simulink model "SiMoDronesMK"  (R2022a)
settings: Solver=FixedStepAuto  StartTime=0.0  StopTime=60  FixedStep=0.005  MaxStep=1e-3  MinStep=5e-5  RelTol=1e-5  AbsTol=1e-5  EnableMultiTasking=on
StopFcn:
  | save log.mat
  | [px4,optitrack,control,simulink]=traite_data_full('log.mat');
  | plot_data;
values from neighbouring files (symbols this model uses):
  aero =     [log.mat]
  drone =     [log.mat]
  dT_px4_udp = 0.02    [SimulationStartupScript.m]    (also in log.mat)
  dT_udp = 0.02    [SimulationStartupScript.m]    (also in log.mat)
  dT_udp_px4 = 0.02    [SimulationStartupScript.m]    (also in log.mat)
  Iload_UAVaxis = [0.00408625  0  0; 0  0.00408625  0; 0  0  8.625e-05]    [log.mat]
  init_state =     [log.mat]
  kpx = 1    [log.mat]
  kvx = 0.35    [log.mat]
  mass = 0.207    [log.mat]
  measure =     [log.mat]
  motor =     [log.mat]
  noisetrigger = 0    [log.mat]
  regul =     [log.mat]
  tdrop = 30    [SimulationStartupScript.m]    (also in log.mat)
  Te = 2e-2    (= 0.02)    [SimulationStartupScript.m]    (also in log.mat)
  th0 = 0.45    [log.mat]
  Ts_px4 = 5e-3    (= 0.005)    [SimulationStartupScript.m]    (also in log.mat)
undefined symbols (not defined in the file or in its folder): DiscIntNeverNeededParam, frame_t, gcbh, sigbuilder_block, sldrt_modeswitch, Standard_Devices, UDP_Protocol
libraries: simulink x11, orocomplib x9, vrlib x5, sldrtlib x4, sharedtransform x3, shared6dofsys x2, sharedutil x1, shared6dof x1, lib_isae_drones x1, simulink_need_slupdate x1, aerolibanimutils x1
(part 3 of 3)

== system SiMoDronesMK/Mass Change Model/Model/Quad rotor model1/Modèle Moments/Calcul Trainée Angulaire ==
  In1 : Inport
  Demux : Demux  Outputs=3
  Demux1 : Demux  Outputs=3
  Gain : Gain  Gain=-1
  Gain2 : Gain  Gain=.5
  Gain3 : Gain  Gain=-1
  Gain4 : Gain  Gain=-1
  Gain5 : Gain  Gain=L
  In2 : InportShadow
  Math Function : Math  Operator=square  SignedPower=on
  Mux2 : Mux  Inputs=3
  Product{1..2,4..5} (4 alike) : Product  RndMeth=Zero
  Product3 : Product  Inputs=3  RndMeth=Zero
  Sign1 : Signum
  Sign2 : Signum
  Sign3 : Signum
  Surface Active : Constant  Value=S_trainee_pqr  SampleTime=0
  density : Constant  Value=rho  SampleTime=0
  dragCoeff : Constant  Value=C_trainee  SampleTime=0
  Out1 : Outport
  wires:
  Surface Active/1 -> Product3/2
  Product3/1 -> Demux/1
  Math Function/1 -> Product4/1
  Gain4/1 -> Mux2/3
  Gain3/1 -> Mux2/2
  Gain/1 -> Mux2/1
  Demux/3 -> Product5/2
  Demux/2 -> Product2/2
  Demux/1 -> Product1/2
  Sign3/1 -> Product5/1
  Sign1/1 -> Product2/1
  Sign2/1 -> Product1/1
  Demux1/3 -> Sign3/1
  Demux1/2 -> Sign1/1
  Demux1/1 -> Sign2/1
  In2/1 -> Demux1/1  "p q r"
  Product1/1 -> Gain/1
  Product2/1 -> Gain3/1
  Product5/1 -> Gain4/1
  density/1 -> Gain2/1
  dragCoeff/1 -> Product3/3  "Cd"
  Product4/1 -> Product3/1
  Gain2/1 -> Product4/2
  In1/1 -> Math Function/1  "p q r"
  Gain5/1 -> Out1/1  "Trainee_angulaires_Rb"
  Mux2/1 -> Gain5/1

== system SiMoDronesMK/Measurement block /Measure /optitrack/XYZ optitrack/1er ordre ==
  x : Inport
  Gain1 : Gain  Gain=1/tr5
  Gain2 : Gain  Gain=K
  Integrator : Integrator  InitialCondition=init_inte
  Sum4 : Sum  Inputs=|+-
  x_retard : Outport
  wires:
  Gain2/1 -> x_retard/1
  x/1 -> Sum4/1
  Sum4/1 -> Gain1/1
  Integrator/1 -> Sum4/2, Gain2/1
  Gain1/1 -> Integrator/1

== system SiMoDronesMK/Measurement block /Measure /optitrack/XYZ optitrack/1er ordre1 ==
  y : Inport
  Gain1 : Gain  Gain=1/tr5
  Gain2 : Gain  Gain=K
  Integrator : Integrator  InitialCondition=init_inte
  Sum4 : Sum  Inputs=|+-
  y_retard : Outport
  wires:
  Gain1/1 -> Integrator/1
  Integrator/1 -> Gain2/1, Sum4/2
  Sum4/1 -> Gain1/1
  y/1 -> Sum4/1
  Gain2/1 -> y_retard/1

== system SiMoDronesMK/Measurement block /Measure /optitrack/XYZ optitrack/1er ordre2 ==
  z : Inport
  Gain1 : Gain  Gain=1/tr5
  Gain2 : Gain  Gain=K
  Integrator : Integrator  InitialCondition=init_inte
  Sum4 : Sum  Inputs=|+-
  z_retard : Outport
  wires:
  Gain2/1 -> z_retard/1
  z/1 -> Sum4/1
  Sum4/1 -> Gain1/1
  Integrator/1 -> Sum4/2, Gain2/1
  Gain1/1 -> Integrator/1

== system SiMoDronesMK/Measurement block /Measure /optitrack/XYZ optitrack/Optitrack  V Noise ==
  Band-Limited White Noise3 : simulink/Sources/Band-Limited White Noise  Cov=[measure.noise_power_vit]  Ts=Te  seed=[23341]
  Constant4 : Constant  Value=noisetrigger  OutDataTypeStr=uint8  SampleTime=Te
  Constant5 : Constant  Value=0  OutDataTypeStr=uint8  SampleTime=Te
  Switch1 : Switch  Criteria=u2 > Threshold  SaturateOnIntegerOverflow=off  InputSameDT=off
  Out1 : Outport
  wires:
  Constant5/1 -> Switch1/3
  Constant4/1 -> Switch1/2
  Switch1/1 -> Out1/1
  Band-Limited White Noise3/1 -> Switch1/1

== system SiMoDronesMK/Measurement block /Measure /optitrack/XYZ optitrack/Optitrack XYZ Noise ==
  Band-Limited White Noise1 : simulink/Sources/Band-Limited White Noise  Cov=[measure.noise_power]  Ts=Te  seed=[23341]
  Constant1 : Constant  Value=noisetrigger  OutDataTypeStr=uint8  SampleTime=Te
  Constant3 : Constant  Value=0  OutDataTypeStr=uint8  SampleTime=Te
  Switch : Switch  Criteria=u2 > Threshold  SaturateOnIntegerOverflow=off  InputSameDT=off
  Out1 : Outport
  wires:
  Switch/1 -> Out1/1
  Constant3/1 -> Switch/3
  Band-Limited White Noise1/1 -> Switch/1
  Constant1/1 -> Switch/2

== system SiMoDronesMK/Measurement block /UDP link + Measure/UDP link/Subsystem4/Float ==
  Float : Inport
  " trame1" : Display  Commented=on
  " trame2" : Display  Commented=on
  Demux : Demux  Outputs=2
  Demux1 : Demux
  MATLAB Function : MATLAB Function  TreatAsAtomicUnit=on
  To Workspace11 : ToWorkspace  VariableName=att_tgt_px4_feedback  SampleTime=Te
  To Workspace4 : ToWorkspace  VariableName=pos_vel_optitrack  SampleTime=Te
  To Workspace6 : ToWorkspace  VariableName=batt_info  SampleTime=Te
  To Workspace7 : ToWorkspace  VariableName=att_eul_px4  SampleTime=Te
  To Workspace8 : ToWorkspace  VariableName=imu_pressure_px4  SampleTime=Te
  To Workspace9 : ToWorkspace  VariableName=att_eul_optitrack  SampleTime=Te
  att_eul_px4 : Outport
  pos_vel_optitrack : Outport  Port=2
  att_eul_optitrack : Outport  Port=3
  tag scope: Vbat=global, pos=global, thrust_back=global
  wires:
  MATLAB Function/2(pos_vel) -> To Workspace4/1, Demux/1, pos_vel_optitrack/1
  MATLAB Function/1(att_eul) -> att_eul_px4/1, To Workspace7/1
  Float/1 -> MATLAB Function/1(u)
  MATLAB Function/3(batt_info) -> To Workspace6/1, [Vbat]
  MATLAB Function/5(att_eul_tgt_out) -> " trame2"/1
  MATLAB Function/4(att_eul_tgt_in) -> " trame1"/1
  Demux/1 -> [pos]
  Demux1/4 -> [thrust_back]
  MATLAB Function/7(att_tgt_PX4) -> Demux1/1, To Workspace11/1
  MATLAB Function/6(optitrack_euler) -> att_eul_optitrack/1, To Workspace9/1
  MATLAB Function/10(imu_acc) -> ?
  MATLAB Function/9(imu_static_pressure) -> To Workspace8/1
  MATLAB Function/8(pos_vel_tgt) -> ?

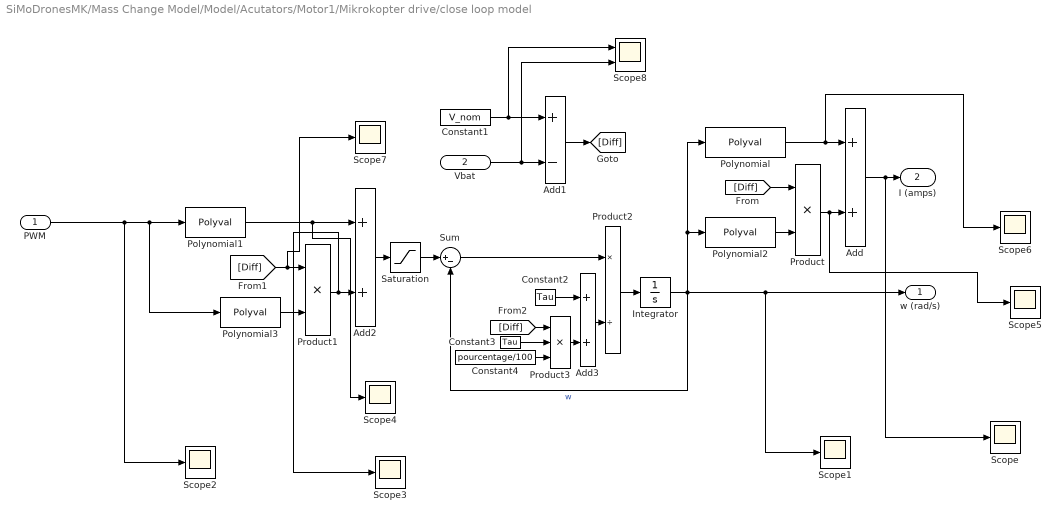
== system SiMoDronesMK/Mass Change Model/Model/Acutators/Motor1/Mikrokopter drive/close loop model ==
  PWM : Inport
  "Vbat " : Inport  Port=2  OutDataTypeStr=double  PortDimensions=1  SampleTime=0
  Add : Sum
  Add1 : Sum  Inputs=+-
  Add2 : Sum
  Add3 : Sum
  Constant1 : Constant  Value=V_nom  SampleTime=-1
  Constant2 : Constant  Value=Tau
  Constant3 : Constant  Value=Tau
  Constant4 : Constant  Value=pourcentage/100
  Integrator : Integrator  InitialCondition=omega_0  LowerSaturationLimit=0
  Polynomial : Polyval  Coefs=coef_w2I
  Polynomial1 : Polyval  Coefs=coef_t2w
  Polynomial2 : Polyval  Coefs=coef_delta_w2I
  Polynomial3 : Polyval  Coefs=coef_delta_t2w
  Product : Product
  Product1 : Product
  Product2 : Product  Inputs=*/
  Product3 : Product  Inputs=***
  Saturation : Saturate  UpperLimit=omega_max  LowerLimit=0
  Scope{,1..7} (8 alike) : Scope
  Scope8 : Scope  NumInputPorts=2
  Sum : Sum  Inputs=|+-
  w (rad/s) : Outport
  I (amps) : Outport  Port=2
  wires:
  Saturation/1 -> Sum/1
  PWM/1 -> Scope2/1, Polynomial1/1, Polynomial3/1
  Integrator/1 -> Scope1/1, w (rad/s)/1, Sum/2, Polynomial2/1, Polynomial/1  "w"
  Sum/1 -> Product2/1
  Polynomial/1 -> Scope6/1, Add/1
  Add/1 -> Scope/1, I (amps)/1
  Add1/1 -> [Diff]
  "Vbat "/1 -> Scope8/2, Add1/2
  Product/1 -> Scope5/1, Add/2
  [Diff] -> Product/1
  Polynomial2/1 -> Product/2
  Polynomial1/1 -> Scope4/1, Add2/1
  Product1/1 -> Scope3/1, Add2/2
  [Diff] -> Scope7/1, Product1/1
  Polynomial3/1 -> Product1/2
  Add2/1 -> Saturation/1
  Product2/1 -> Integrator/1
  Add3/1 -> Product2/2
  Constant2/1 -> Add3/1
  Product3/1 -> Add3/2
  [Diff] -> Product3/1
  Constant3/1 -> Product3/2
  Constant4/1 -> Product3/3
  Constant1/1 -> Scope8/1, Add1/1

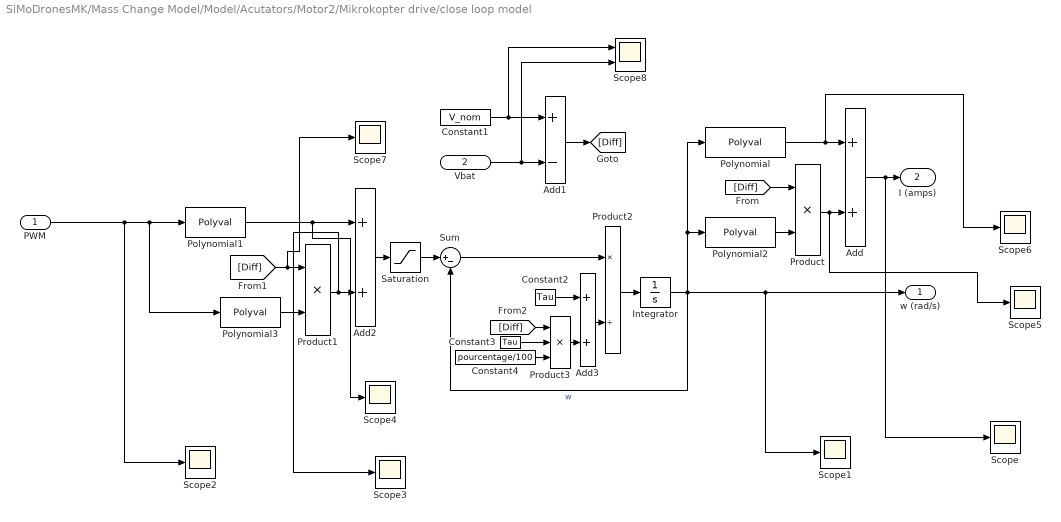
== system SiMoDronesMK/Mass Change Model/Model/Acutators/Motor2/Mikrokopter drive/close loop model ==
  PWM : Inport
  "Vbat " : Inport  Port=2  OutDataTypeStr=double  PortDimensions=1  SampleTime=0
  Add : Sum
  Add1 : Sum  Inputs=+-
  Add2 : Sum
  Add3 : Sum
  Constant1 : Constant  Value=V_nom  SampleTime=-1
  Constant2 : Constant  Value=Tau
  Constant3 : Constant  Value=Tau
  Constant4 : Constant  Value=pourcentage/100
  Integrator : Integrator  InitialCondition=omega_0  LowerSaturationLimit=0
  Polynomial : Polyval  Coefs=coef_w2I
  Polynomial1 : Polyval  Coefs=coef_t2w
  Polynomial2 : Polyval  Coefs=coef_delta_w2I
  Polynomial3 : Polyval  Coefs=coef_delta_t2w
  Product : Product
  Product1 : Product
  Product2 : Product  Inputs=*/
  Product3 : Product  Inputs=***
  Saturation : Saturate  UpperLimit=omega_max  LowerLimit=0
  Scope{,1..7} (8 alike) : Scope
  Scope8 : Scope  NumInputPorts=2
  Sum : Sum  Inputs=|+-
  w (rad/s) : Outport
  I (amps) : Outport  Port=2
  wires:
  Saturation/1 -> Sum/1
  PWM/1 -> Scope2/1, Polynomial1/1, Polynomial3/1
  Integrator/1 -> Scope1/1, w (rad/s)/1, Sum/2, Polynomial2/1, Polynomial/1  "w"
  Sum/1 -> Product2/1
  Polynomial/1 -> Scope6/1, Add/1
  Add/1 -> Scope/1, I (amps)/1
  Add1/1 -> [Diff]
  "Vbat "/1 -> Scope8/2, Add1/2
  Product/1 -> Scope5/1, Add/2
  [Diff] -> Product/1
  Polynomial2/1 -> Product/2
  Polynomial1/1 -> Scope4/1, Add2/1
  Product1/1 -> Scope3/1, Add2/2
  [Diff] -> Scope7/1, Product1/1
  Polynomial3/1 -> Product1/2
  Add2/1 -> Saturation/1
  Product2/1 -> Integrator/1
  Add3/1 -> Product2/2
  Constant2/1 -> Add3/1
  Product3/1 -> Add3/2
  [Diff] -> Product3/1
  Constant3/1 -> Product3/2
  Constant4/1 -> Product3/3
  Constant1/1 -> Scope8/1, Add1/1

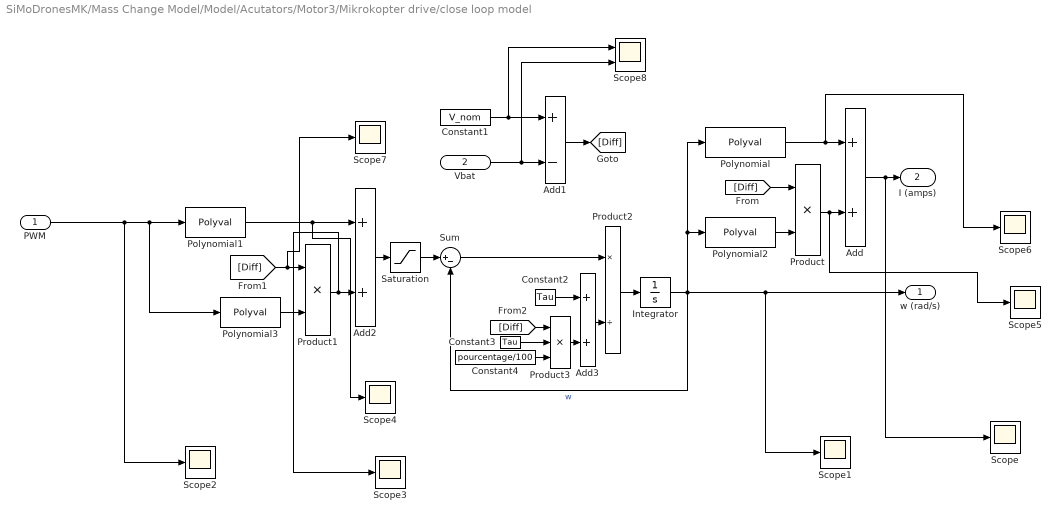
== system SiMoDronesMK/Mass Change Model/Model/Acutators/Motor3/Mikrokopter drive/close loop model ==
  PWM : Inport
  "Vbat " : Inport  Port=2  OutDataTypeStr=double  PortDimensions=1  SampleTime=0
  Add : Sum
  Add1 : Sum  Inputs=+-
  Add2 : Sum
  Add3 : Sum
  Constant1 : Constant  Value=V_nom  SampleTime=-1
  Constant2 : Constant  Value=Tau
  Constant3 : Constant  Value=Tau
  Constant4 : Constant  Value=pourcentage/100
  Integrator : Integrator  InitialCondition=omega_0  LowerSaturationLimit=0
  Polynomial : Polyval  Coefs=coef_w2I
  Polynomial1 : Polyval  Coefs=coef_t2w
  Polynomial2 : Polyval  Coefs=coef_delta_w2I
  Polynomial3 : Polyval  Coefs=coef_delta_t2w
  Product : Product
  Product1 : Product
  Product2 : Product  Inputs=*/
  Product3 : Product  Inputs=***
  Saturation : Saturate  UpperLimit=omega_max  LowerLimit=0
  Scope{,1..7} (8 alike) : Scope
  Scope8 : Scope  NumInputPorts=2
  Sum : Sum  Inputs=|+-
  w (rad/s) : Outport
  I (amps) : Outport  Port=2
  wires:
  Saturation/1 -> Sum/1
  PWM/1 -> Scope2/1, Polynomial1/1, Polynomial3/1
  Integrator/1 -> Scope1/1, w (rad/s)/1, Sum/2, Polynomial2/1, Polynomial/1  "w"
  Sum/1 -> Product2/1
  Polynomial/1 -> Scope6/1, Add/1
  Add/1 -> Scope/1, I (amps)/1
  Add1/1 -> [Diff]
  "Vbat "/1 -> Scope8/2, Add1/2
  Product/1 -> Scope5/1, Add/2
  [Diff] -> Product/1
  Polynomial2/1 -> Product/2
  Polynomial1/1 -> Scope4/1, Add2/1
  Product1/1 -> Scope3/1, Add2/2
  [Diff] -> Scope7/1, Product1/1
  Polynomial3/1 -> Product1/2
  Add2/1 -> Saturation/1
  Product2/1 -> Integrator/1
  Add3/1 -> Product2/2
  Constant2/1 -> Add3/1
  Product3/1 -> Add3/2
  [Diff] -> Product3/1
  Constant3/1 -> Product3/2
  Constant4/1 -> Product3/3
  Constant1/1 -> Scope8/1, Add1/1

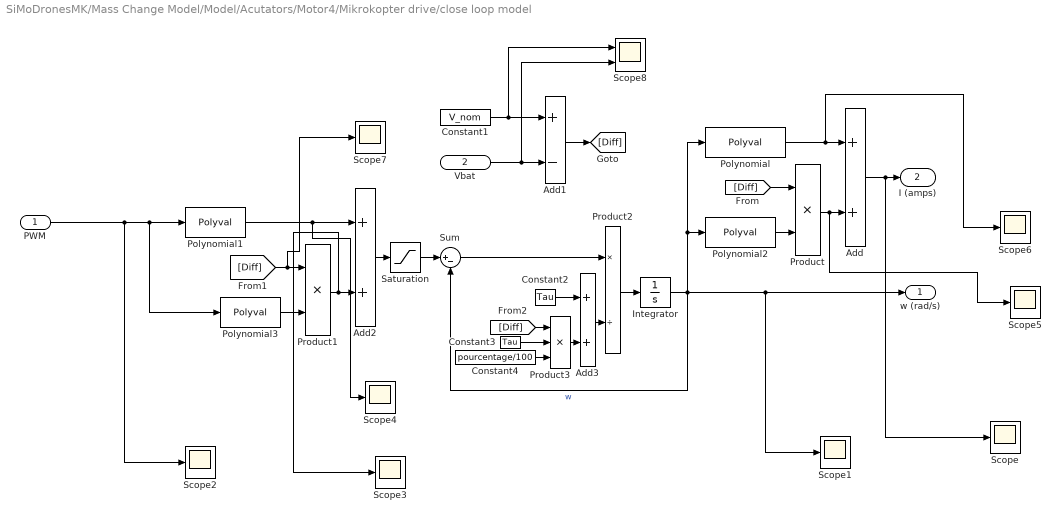
== system SiMoDronesMK/Mass Change Model/Model/Acutators/Motor4/Mikrokopter drive/close loop model ==
  PWM : Inport
  "Vbat " : Inport  Port=2  OutDataTypeStr=double  PortDimensions=1  SampleTime=0
  Add : Sum
  Add1 : Sum  Inputs=+-
  Add2 : Sum
  Add3 : Sum
  Constant1 : Constant  Value=V_nom  SampleTime=-1
  Constant2 : Constant  Value=Tau
  Constant3 : Constant  Value=Tau
  Constant4 : Constant  Value=pourcentage/100
  Integrator : Integrator  InitialCondition=omega_0  LowerSaturationLimit=0
  Polynomial : Polyval  Coefs=coef_w2I
  Polynomial1 : Polyval  Coefs=coef_t2w
  Polynomial2 : Polyval  Coefs=coef_delta_w2I
  Polynomial3 : Polyval  Coefs=coef_delta_t2w
  Product : Product
  Product1 : Product
  Product2 : Product  Inputs=*/
  Product3 : Product  Inputs=***
  Saturation : Saturate  UpperLimit=omega_max  LowerLimit=0
  Scope{,1..7} (8 alike) : Scope
  Scope8 : Scope  NumInputPorts=2
  Sum : Sum  Inputs=|+-
  w (rad/s) : Outport
  I (amps) : Outport  Port=2
  wires:
  Saturation/1 -> Sum/1
  PWM/1 -> Scope2/1, Polynomial1/1, Polynomial3/1
  Integrator/1 -> Scope1/1, w (rad/s)/1, Sum/2, Polynomial2/1, Polynomial/1  "w"
  Sum/1 -> Product2/1
  Polynomial/1 -> Scope6/1, Add/1
  Add/1 -> Scope/1, I (amps)/1
  Add1/1 -> [Diff]
  "Vbat "/1 -> Scope8/2, Add1/2
  Product/1 -> Scope5/1, Add/2
  [Diff] -> Product/1
  Polynomial2/1 -> Product/2
  Polynomial1/1 -> Scope4/1, Add2/1
  Product1/1 -> Scope3/1, Add2/2
  [Diff] -> Scope7/1, Product1/1
  Polynomial3/1 -> Product1/2
  Add2/1 -> Saturation/1
  Product2/1 -> Integrator/1
  Add3/1 -> Product2/2
  Constant2/1 -> Add3/1
  Product3/1 -> Add3/2
  [Diff] -> Product3/1
  Constant3/1 -> Product3/2
  Constant4/1 -> Product3/3
  Constant1/1 -> Scope8/1, Add1/1

== matlab function SiMoDronesMK/Attitude control/Inner Loop (PX4)/Attitude Control Actuators (PID-PX4)/Régulations/PX4_attitude_control ==
  data: t input; att_sp_RBod input; rates_sp output; att_RBod input; param_att_p input; mc_rate_min input; mc_rate_max input; yaw_sp_move_rate input; yaw_ff input
function rates_sp = PX4_attitude_control(t, att_sp_RBod, att_RBod, param_att_p, mc_rate_min, mc_rate_max, yaw_sp_move_rate, yaw_ff)
%#codegen
coder.extrinsic('warning')
coder.extrinsic('num2str')

% construct attitude setpoint rotation matrix %
R_sp = att_sp_RBod';

% rotation matrix for current state %
R = att_RBod';

% all input data is ready, run controller itself %

% try to move thrust vector shortest way, because yaw response is slower than roll/pitch %
R_z = R(:,3);
R_sp_z = R_sp(:,3);

% axis and sin(angle) of desired rotation %
e_R = transpose(R) * (cross(R_z,R_sp_z));

% calculate angle error %
e_R_z_sin = norm(e_R);
e_R_z_cos = dot(R_z,R_sp_z);

% calculate weight for yaw control %
yaw_w = R_sp(3, 3) * R_sp(3, 3);

% calculate rotation matrix after roll/pitch only rotation %

if (e_R_z_sin > 0.0)
    % get axis-angle representation %
    e_R_z_angle = atan2(e_R_z_sin, e_R_z_cos);
    e_R_z_axis = e_R / e_R_z_sin;
    
    e_R = e_R_z_axis * e_R_z_angle;
    
    % cross product matrix for e_R_axis %
    e_R_cp = zeros(3,3);
    e_R_cp(1, 2) = -e_R_z_axis(3);
    e_R_cp(1, 3) = e_R_z_axis(2);
    e_R_cp(2, 1) = e_R_z_axis(3);
    e_R_cp(2, 3) = -e_R_z_axis(1);
    e_R_cp(3, 1) = -e_R_z_axis(2);
    e_R_cp(3, 2) = e_R_z_axis(1);
    
    % rotation matrix for roll/pitch only rotation %
    R_rp = R * (eye(3) + e_R_cp * e_R_z_sin + e_R_cp * e_R_cp * (1.0 - e_R_z_cos));
    
else
    % zero roll/pitch rotation %
    R_rp = R;
    warning(['zero roll/pitch rotation at time: ' num2str(t)])
end

% R_rp and R_sp have the same Z axis, calculate yaw error %
R_sp_x = R_sp(:,1);
R_rp_x = R_rp(:,1);
e_R(3) = atan2(dot(cross(R_rp_x, R_sp_x), R_sp_z), dot(R_rp_x, R_sp_x)) * yaw_w;

if (e_R_z_cos < 0.0)
    % for large thrust vector rotations use another rotation method:
    % calculate angle and axis for R -> R_sp rotation directly %
    
    q = dcm2quat_simulink(transpose(R) * R_sp);
    e_R_d = q(2:4)';
    e_R_d = e_R_d/norm(e_R_d);
    e_R_d = e_R_d *(2 * atan2(norm(e_R_d), q(1)));
    
    % use fusion of Z axis based rotation and direct rotation %
    direct_w = e_R_z_cos * e_R_z_cos * yaw_w;
    e_R = e_R * (1 - direct_w) + e_R_d * direct_w;
    warning(['large thrust error at time: ' num2str(t)])
end

% calculate angular rates setpoint %
rates_sp = param_att_p .* e_R;

% limit rates %
for i = 1:3
    if rates_sp(i) > mc_rate_max(i)
        rates_sp(i) = mc_rate_max(i);
    end
    if rates_sp(i) < mc_rate_min(i)
        rates_sp(i) = mc_rate_min(i);
    end
end

% feed forward yaw setpoint rate %
rates_sp(3) =  rates_sp(3) + yaw_sp_move_rate * yaw_w * yaw_ff;



function q = dcm2quat_simulink( dcm )
%  DCM2QUAT Convert direction cosine matrix to quaternion.
%   Q = DCM2QUAT( N ) calculates the quaternion, Q, for given
%   direction cosine matrix, N.   Input N is a 3-by-3-by-M matrix of
%   orthogonal direction cosine matrices.  The direction cosine matrix performs the
%   coordinate transformation of a vector in inertial axes to a vector in
%   body axes.  Q returns an M-by-4 matrix containing M quaternions. Q has
%   its scalar number as the first column.
%
%   Examples:
%
%   Determine the quaternion from direction cosine matrix:
%      dcm = [0 1 0; 1 0 0; 0 0 1];
%      q = dcm2quat(dcm)
%
%   Determine the quaternions from multiple direction cosine matrices:
%      dcm        = [ 0 1 0; 1 0 0; 0 0 1];
%      dcm(:,:,2) = [ 0.4330    0.2500   -0.8660; ...
%                     0.1768    0.9186    0.3536; ...
%                     0.8839   -0.3062    0.3536];
%      q = dcm2quat(dcm)
%
%   See also ANGLE2DCM, DCM2ANGLE, QUAT2DCM, QUAT2ANGLE, ANGLE2QUAT.

%   Copyright 2000-2010 The MathWorks, Inc.

if any(~isreal(dcm) || ~isnumeric(dcm))
    error(message('aero:dcm2quat:isNotReal'));
end

if ((size(dcm,1) ~= 3) || (size(dcm,2) ~= 3))
    error(message('aero:dcm2quat:wrongDimension'));
end

q = zeros(size(dcm,3),4);

for i = size(dcm,3):-1:1
    
    q(i,4) =  0;
    
    tr = trace(dcm(:,:,i));
    
    if (tr > 0)
        sqtrp1 = sqrt( tr + 1.0 );
        
        q(i,1) = 0.5*sqtrp1;
        q(i,2) = (dcm(2, 3, i) - dcm(3, 2, i))/(2.0*sqtrp1);
        q(i,3) = (dcm(3, 1, i) - dcm(1, 3, i))/(2.0*sqtrp1);
        q(i,4) = (dcm(1, 2, i) - dcm(2, 1, i))/(2.0*sqtrp1);
    else
        d = diag(dcm(:,:,i));
        if ((d(2) > d(1)) && (d(2) > d(3)))
            % max value at dcm(2,2,i)
            sqdip1 = sqrt(d(2) - d(1) - d(3) + 1.0 );
            
            q(i,3) = 0.5*sqdip1;
            
            if ( sqdip1 ~= 0 )
                sqdip1 = 0.5/sqdip1;
            end
            
            q(i,1) = (dcm(3, 1, i) - dcm(1, 3, i))*sqdip1;
            q(i,2) = (dcm(1, 2, i) + dcm(2, 1, i))*sqdip1;
            q(i,4) = (dcm(2, 3, i) + dcm(3, 2, i))*sqdip1;
        elseif (d(3) > d(1))
            % max value at dcm(3,3,i)
            sqdip1 = sqrt(d(3) - d(1) - d(2) + 1.0 );
            
            q(i,4) = 0.5*sqdip1;
            
            if ( sqdip1 ~= 0 )
                sqdip1 = 0.5/sqdip1;
            end
            
            q(i,1) = (dcm(1, 2, i) - dcm(2, 1, i))*sqdip1;
            q(i,2) = (dcm(3, 1, i) + dcm(1, 3, i))*sqdip1;
            q(i,3) = (dcm(2, 3, i) + dcm(3, 2, i))*sqdip1;
        else
            % max value at dcm(1,1,i)
            sqdip1 = sqrt(d(1) - d(2) - d(3) + 1.0 );
            
            q(i,2) = 0.5*sqdip1;
            
            if ( sqdip1 ~= 0 )
                sqdip1 = 0.5/sqdip1;
            end
            
            q(i,1) = (dcm(2, 3, i) - dcm(3, 2, i))*sqdip1;
            q(i,3) = (dcm(1, 2, i) + dcm(2, 1, i))*sqdip1;
            q(i,4) = (dcm(3, 1, i) + dcm(1, 3, i))*sqdip1;
        end
    end
end

== matlab function SiMoDronesMK/Attitude control/Inner Loop (PX4)/Attitude Control Actuators (PID-PX4)/Régulations/PX4_attitude_rate ==
  data: t input; rates_sp input; rates input; params_rate_p input; params_rate_i input; params_rate_d input; params_rate_ff input; att_control output
function att_control = PX4_attitude_control(t, rates_sp, rates, params_rate_p, params_rate_i, params_rate_d,...
    params_rate_ff)
%#codegen

persistent rates_int t_av rates_prev rates_sp_prev

% reset integral at start */
if isempty(rates_int)
    t_av=-0.01;
    rates_int = zeros(3,1);
    rates_prev = zeros(3,1);
    rates_sp_prev = zeros(3,1);
end

dt=t-t_av;
t_av=t;

% angular rates error */
rates_err = rates_sp - rates;

att_control = zeros(3,1);
for i=1:3
    att_control(i) = params_rate_p(i)*rates_err(i) + ...
    params_rate_d(i)*(rates_prev(i) - rates(i))/dt + ...
    rates_int(i) + ...
    params_rate_ff(i)*(rates_sp(i) - rates_sp_prev(i))/dt;
end

rates_sp_prev = rates_sp;
rates_prev = rates;

% update integral only if not saturated on low limit and if motor commands are not saturated */
% if (v_att_sp_thrust > min_takeoff_thrust)
%     
%     for i=1:3
%         
%         if (abs(att_control(i)) < v_att_sp_thrust)
%             
            rate_i = rates_int(i) + params_rate_i(i) * rates_err(i) * dt;
            rates_int(i) = rate_i;
%         end
%     end
% end

end

== matlab function SiMoDronesMK/Measurement block /UDP link + Measure/UDP link/Subsystem4/Float/MATLAB Function ==
  data: u input; att_eul output; pos_vel output; batt_info output; att_eul_tgt_in output; att_eul_tgt_out output; optitrack_euler output; att_tgt_PX4 output; pos_vel_tgt output; imu_static_pressure output; imu_acc output
function [att_eul, pos_vel, batt_info, att_eul_tgt_in, ...
    att_eul_tgt_out, ... optitrack_quat,
    optitrack_euler, ...
    att_tgt_PX4, pos_vel_tgt, imu_static_pressure, imu_acc...
    ] = UnpackMorseFloats(u)
%#codegen

% attitude_euler
i = 0; % start index in the c++ code
att_eul = [u(i+1);u(i+2);u(i+3);u(i+4);u(i+5);u(i+6)];

% pos_vel, ENU to NED
i = 6; % start index in the c++ code
pos_vel = [u(i+1);u(i+2);u(i+3);u(i+4);u(i+5);u(i+6)].*[1;-1;-1;1;-1;-1];

% batt_info
i = 12; % start index in the c++ code
batt_info = [u(i+1);u(i+2);u(i+3)];

% attitude__target_in
i = 20; % start index in the c++ code
att_eul_tgt_in = [u(i+1);u(i+2);u(i+3);u(i+4);u(i+5)];

% attitude__target_out
i = 25; % start index in the c++ code
att_eul_tgt_out = [u(i+1);u(i+2);u(i+3);u(i+4);u(i+5)];

% attitude target feedback from PX4
i = 30; % start index in the c++ code
att_tgt_PX4 = [u(i+1);u(i+2);u(i+3);u(i+4)];

% optitrack_eul
i = 34; % start index in the c++ code
optitrack_euler = [u(i+1);u(i+2);u(i+3);u(i+4);u(i+5);u(i+6)];

% pos_vel target
i = 40; % start index in the c++ code
pos_vel_tgt = [u(i+1);u(i+2);u(i+3);u(i+4);u(i+5);u(i+6)];

% accel output from embedded guidance
i = 46; % start index in the c++ code
imu_acc = [u(i+1);u(i+2);u(i+3)];

% pression output from embedded guidance
i = 49; % start index in the c++ code
imu_static_pressure = u(i+1);

== matlab function SiMoDronesMK/Measurement block /UDP link + Measure/UDP link/Subsystem4/MATLAB Function ==
  data: u input; ramp_feedback output; offboard_button output; motor_speed output; servo output
function [ramp_feedback, offboard_button,motor_speed,servo] = UnpackMorseIntegers(u)
%#codegen

% ramp feedback
i = 0; % start index in the c++ code
ramp_feedback = u(i+1);


% offboard button feedback
i = 1; % start index in the c++ code
offboard_button = u(i+1);

% Servos (8 outputs)
i=21;
motor_speed = [u(i+1);u(i+2);u(i+3);u(i+4)];
servo = u(i+5);

== matlab function SiMoDronesMK/Attitude control/Udp send/udpSend ==
  data: att_eul_tgt input Bus: attitude_target; floats output single size=50; simulink_out_mode input; integers output int16 size=50; ramp input; simulink_activated input
function [floats,integers] = udpSend(att_eul_tgt, simulink_out_mode, ramp, simulink_activated)
%#codegen

floats = single(zeros(50,1));
integers = zeros(50,1);

floats(0+1) = att_eul_tgt.roll;
floats(1+1) = att_eul_tgt.pitch;
floats(2+1) = att_eul_tgt.yaw;
floats(3+1) = att_eul_tgt.thrust;

% simulink_mode, if 1 output simulink tgt, if 0 output tgt input
integers(0+1) = simulink_out_mode;

% output ramp to measure transmission delay
integers(1+1) = ramp;

% simulink_output_activated
integers(2+1) = simulink_activated;

integers = int16(integers);

== matlab function SiMoDronesMK/Measurement block /Measure /optitrack/Attitude optitrack/MATLAB Function ==
  data: in input; out output
function out = fcn(in)
%#codegen

%y = mod(u+pi, 2*pi) - pi;

if (in < -pi) || (pi < in)
    out = in + pi;
    out = mod(out, 2*pi) - pi;
else
    out = in;
end

== matlab function SiMoDronesMK/Measurement block /Measure /px4/MATLAB Function1 ==
  data: in input; out output
function out = fcn(in)
%#codegen

%y = mod(u+pi, 2*pi) - pi;

if (in < -pi) || (pi < in)
    out = in + pi;
    out = mod(out, 2*pi) - pi;
else
    out = in;
end
